simulink model "InvertedPendulum"  (R2020b)
settings: Solver=VariableStepAuto  StartTime=0.0  StopTime=tm  RelTol=1e-3
values from neighbouring files (symbols this model uses):
  A = [0,1,0,0; 0,a1,0,0; 0,0,0,1; 0,a2,a3,0]    [InvertedPendulumC.m]
  B = [0,b1,0,b2]'    [InvertedPendulumC.m]
  C = [1,0,0,0; 0,0,1,0]    [InvertedPendulumC.m]
  K = place(A,B,P)    [InvertedPendulumC.m]
settings Model: Creator=huang  LastModifiedBy=huang

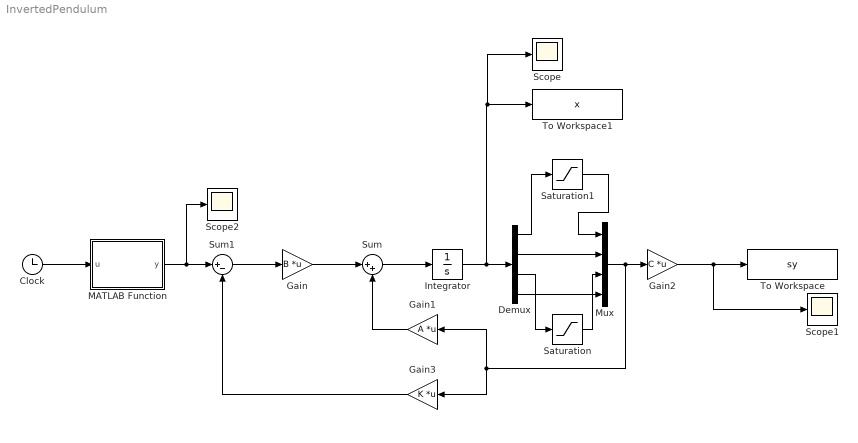
== system InvertedPendulum ==
  Clock : Clock
  Demux : Demux
  Gain : Gain  Gain=B  Multiplication=Matrix(K*u)
  Gain1 : Gain  Gain=A  Multiplication=Matrix(K*u)
  Gain2 : Gain  Gain=C  Multiplication=Matrix(K*u)
  Gain3 : Gain  Gain=K  Multiplication=Matrix(K*u)
  Integrator : Integrator
  MATLAB Function : MATLAB Function  TreatAsAtomicUnit=on
  Mux : Mux
  Saturation : Saturate  UpperLimit=pi/2  LowerLimit=-pi/2
  Saturation1 : Saturate
  Scope : Scope
  Scope1 : Scope
  Scope2 : Scope
  Sum : Sum  Inputs=|++
  Sum1 : Sum  Inputs=|+-
  To Workspace : ToWorkspace  VariableName=sy  SampleTime=-1
      settings: Save2DSignal=2-D array (concatenate along first dimension)
  To Workspace1 : ToWorkspace  VariableName=x  SampleTime=-1
      settings: Save2DSignal=2-D array (concatenate along first dimension)
  wires:
  Gain/1 -> Sum/1
  Sum/1 -> Integrator/1
  Gain1/1 -> Sum/2
  Gain2/1 -> Scope1/1, To Workspace/1
  Sum1/1 -> Gain/1
  Clock/1 -> MATLAB Function/1(u)
  Integrator/1 -> Demux/1, Scope/1, To Workspace1/1
  MATLAB Function/1(y) -> Scope2/1, Sum1/1
  Demux/2 -> Mux/2
  Demux/4 -> Mux/4
  Demux/3 -> Saturation/1
  Saturation/1 -> Mux/3
  Mux/1 -> Gain1/1, Gain3/1, Gain2/1
  Demux/1 -> Saturation1/1
  Saturation1/1 -> Mux/1
  Gain3/1 -> Sum1/2

== matlab function InvertedPendulum/MATLAB Function ==
  data: u input; y output
function y = fcn(u)
    ts=0.001;
    h=5/ts;
    if(u<ts)
        y=h;
    else
        y=0;
    end
end
